simulink library "TYPEA_MASTER"  (Simulink 8.6)
settings: Solver=ode45  StartTime=0.0  StopTime=10.0  RelTol=1e-3
undefined symbols (not defined in the file): CRYP_OLSERVO, PAY_OLSERVO
libraries: cdsFilt x12, GAS_MODAL_MASTER x8, cdsEpicsBinIn x6, VIS_LIB x5, cdsEpicsOut x4, BIO_TYPEA_MASTER x3, cdsDacKill x3, ADV_BF_MASTER x2, cdsEpicsStringIn x2, TYPEA_GAS_MODAL_MASTER x2, ISC_common x2, CRYP_IM_MASTER x2
(part 2 of 2)

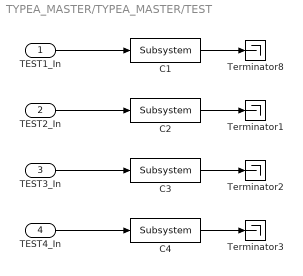
== system TYPEA_MASTER/TYPEA_MASTER/TEST ==
  TEST1_In : Inport
  TEST2_In : Inport  Port=2
  TEST3_In : Inport  Port=3
  TEST4_In : Inport  Port=4
  C1 : cdsFilt/Subsystem  Tag=cdsFilt  Description=|
      | Purpose:                                                                                                                                                                                                                                  
      | Standard CDS IIR filter module.                                                                                                                                                                                                           
      |                                                                                                                                                                                                                                           
      | Operation:                                                                                                                                                                                                                                
      | Consists of 10 second order section IIR filters, plus a ramped gain stage. In FE code, also provides pre-defined test points and excitation channel inputs. The filter coefficients are defined in the LIGO system using the 'foton' tool.
      |                                                                                                                                                                                                                                           
      | Usage:                                                                                                                                                                                                                                    
      | Name the part with the desired filter module name.
      settings: AttributesFormatString=%<Tag>
  C2 : cdsFilt/Subsystem  Tag=cdsFilt  Description=|
      | Purpose:                                                                                                                                                                                                                                  
      | Standard CDS IIR filter module.                                                                                                                                                                                                           
      |                                                                                                                                                                                                                                           
      | Operation:                                                                                                                                                                                                                                
      | Consists of 10 second order section IIR filters, plus a ramped gain stage. In FE code, also provides pre-defined test points and excitation channel inputs. The filter coefficients are defined in the LIGO system using the 'foton' tool.
      |                                                                                                                                                                                                                                           
      | Usage:                                                                                                                                                                                                                                    
      | Name the part with the desired filter module name.
      settings: AttributesFormatString=%<Tag>
  C3 : cdsFilt/Subsystem  Tag=cdsFilt  Description=|
      | Purpose:                                                                                                                                                                                                                                  
      | Standard CDS IIR filter module.                                                                                                                                                                                                           
      |                                                                                                                                                                                                                                           
      | Operation:                                                                                                                                                                                                                                
      | Consists of 10 second order section IIR filters, plus a ramped gain stage. In FE code, also provides pre-defined test points and excitation channel inputs. The filter coefficients are defined in the LIGO system using the 'foton' tool.
      |                                                                                                                                                                                                                                           
      | Usage:                                                                                                                                                                                                                                    
      | Name the part with the desired filter module name.
      settings: AttributesFormatString=%<Tag>
  C4 : cdsFilt/Subsystem  Tag=cdsFilt  Description=|
      | Purpose:                                                                                                                                                                                                                                  
      | Standard CDS IIR filter module.                                                                                                                                                                                                           
      |                                                                                                                                                                                                                                           
      | Operation:                                                                                                                                                                                                                                
      | Consists of 10 second order section IIR filters, plus a ramped gain stage. In FE code, also provides pre-defined test points and excitation channel inputs. The filter coefficients are defined in the LIGO system using the 'foton' tool.
      |                                                                                                                                                                                                                                           
      | Usage:                                                                                                                                                                                                                                    
      | Name the part with the desired filter module name.
      settings: AttributesFormatString=%<Tag>
  Terminator{1..3,8} (4 alike) : Terminator
  wires:
  C2/1 -> Terminator1/1
  C3/1 -> Terminator2/1
  C1/1 -> Terminator8/1
  C4/1 -> Terminator3/1
  TEST1_In/1 -> C1/1
  TEST2_In/1 -> C2/1
  TEST3_In/1 -> C3/1
  TEST4_In/1 -> C4/1

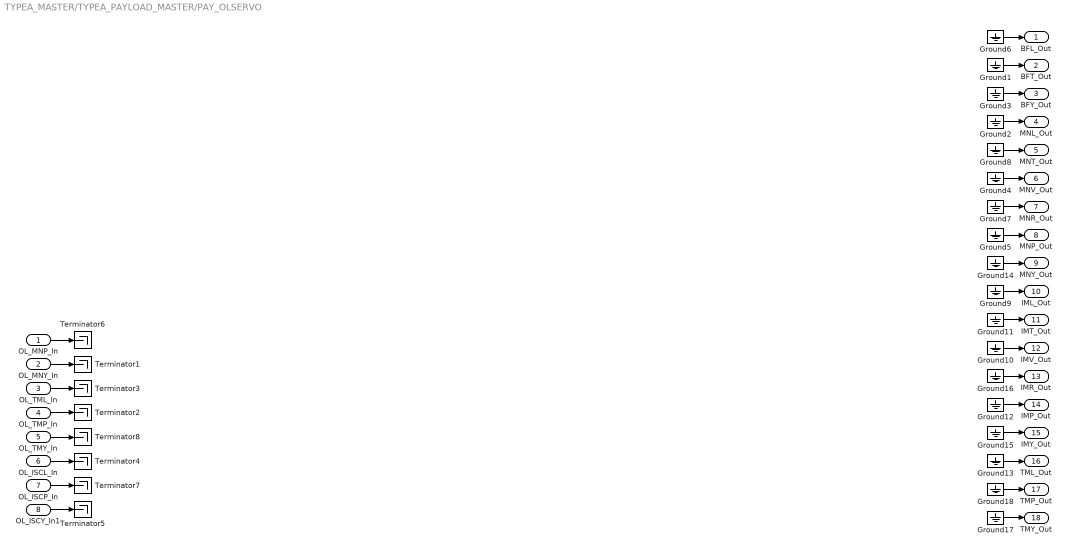
== system TYPEA_MASTER/TYPEA_PAYLOAD_MASTER/PAY_OLSERVO ==
  OL_MNP_In : Inport
  OL_MNY_In : Inport  Port=2
  OL_TML_In : Inport  Port=3
  OL_TMP_In : Inport  Port=4
  OL_TMY_In : Inport  Port=5
  OL_ISCL_In : Inport  Port=6
  OL_ISCP_In : Inport  Port=7
  OL_ISCY_In1 : Inport  Port=8
  Ground{1..18} (18 alike) : Ground
  Terminator{1..8} (8 alike) : Terminator
  BFL_Out : Outport
  BFT_Out : Outport  Port=2
  BFY_Out : Outport  Port=3
  MNL_Out : Outport  Port=4
  MNT_Out : Outport  Port=5
  MNV_Out : Outport  Port=6
  MNR_Out : Outport  Port=7
  MNP_Out : Outport  Port=8
  MNY_Out : Outport  Port=9
  IML_Out : Outport  Port=10
  IMT_Out : Outport  Port=11
  IMV_Out : Outport  Port=12
  IMR_Out : Outport  Port=13
  IMP_Out : Outport  Port=14
  IMY_Out : Outport  Port=15
  TML_Out : Outport  Port=16
  TMP_Out : Outport  Port=17
  TMY_Out : Outport  Port=18
  wires:
  Ground6/1 -> BFL_Out/1
  OL_MNP_In/1 -> Terminator6/1
  OL_MNY_In/1 -> Terminator1/1
  OL_TML_In/1 -> Terminator3/1
  OL_TMP_In/1 -> Terminator2/1
  OL_TMY_In/1 -> Terminator8/1
  OL_ISCL_In/1 -> Terminator4/1
  OL_ISCP_In/1 -> Terminator7/1
  OL_ISCY_In1/1 -> Terminator5/1
  Ground1/1 -> BFT_Out/1
  Ground3/1 -> BFY_Out/1
  Ground2/1 -> MNL_Out/1
  Ground8/1 -> MNT_Out/1
  Ground4/1 -> MNV_Out/1
  Ground7/1 -> MNR_Out/1
  Ground5/1 -> MNP_Out/1
  Ground14/1 -> MNY_Out/1
  Ground9/1 -> IML_Out/1
  Ground11/1 -> IMT_Out/1
  Ground10/1 -> IMV_Out/1
  Ground16/1 -> IMR_Out/1
  Ground12/1 -> IMP_Out/1
  Ground15/1 -> IMY_Out/1
  Ground13/1 -> TML_Out/1
  Ground18/1 -> TMP_Out/1
  Ground17/1 -> TMY_Out/1

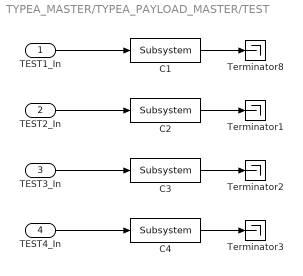
== system TYPEA_MASTER/TYPEA_PAYLOAD_MASTER/TEST ==
  TEST1_In : Inport
  TEST2_In : Inport  Port=2
  TEST3_In : Inport  Port=3
  TEST4_In : Inport  Port=4
  C1 : cdsFilt/Subsystem  Tag=cdsFilt  Description=|
      | Purpose:                                                                                                                                                                                                                                  
      | Standard CDS IIR filter module.                                                                                                                                                                                                           
      |                                                                                                                                                                                                                                           
      | Operation:                                                                                                                                                                                                                                
      | Consists of 10 second order section IIR filters, plus a ramped gain stage. In FE code, also provides pre-defined test points and excitation channel inputs. The filter coefficients are defined in the LIGO system using the 'foton' tool.
      |                                                                                                                                                                                                                                           
      | Usage:                                                                                                                                                                                                                                    
      | Name the part with the desired filter module name.
      settings: AttributesFormatString=%<Tag>
  C2 : cdsFilt/Subsystem  Tag=cdsFilt  Description=|
      | Purpose:                                                                                                                                                                                                                                  
      | Standard CDS IIR filter module.                                                                                                                                                                                                           
      |                                                                                                                                                                                                                                           
      | Operation:                                                                                                                                                                                                                                
      | Consists of 10 second order section IIR filters, plus a ramped gain stage. In FE code, also provides pre-defined test points and excitation channel inputs. The filter coefficients are defined in the LIGO system using the 'foton' tool.
      |                                                                                                                                                                                                                                           
      | Usage:                                                                                                                                                                                                                                    
      | Name the part with the desired filter module name.
      settings: AttributesFormatString=%<Tag>
  C3 : cdsFilt/Subsystem  Tag=cdsFilt  Description=|
      | Purpose:                                                                                                                                                                                                                                  
      | Standard CDS IIR filter module.                                                                                                                                                                                                           
      |                                                                                                                                                                                                                                           
      | Operation:                                                                                                                                                                                                                                
      | Consists of 10 second order section IIR filters, plus a ramped gain stage. In FE code, also provides pre-defined test points and excitation channel inputs. The filter coefficients are defined in the LIGO system using the 'foton' tool.
      |                                                                                                                                                                                                                                           
      | Usage:                                                                                                                                                                                                                                    
      | Name the part with the desired filter module name.
      settings: AttributesFormatString=%<Tag>
  C4 : cdsFilt/Subsystem  Tag=cdsFilt  Description=|
      | Purpose:                                                                                                                                                                                                                                  
      | Standard CDS IIR filter module.                                                                                                                                                                                                           
      |                                                                                                                                                                                                                                           
      | Operation:                                                                                                                                                                                                                                
      | Consists of 10 second order section IIR filters, plus a ramped gain stage. In FE code, also provides pre-defined test points and excitation channel inputs. The filter coefficients are defined in the LIGO system using the 'foton' tool.
      |                                                                                                                                                                                                                                           
      | Usage:                                                                                                                                                                                                                                    
      | Name the part with the desired filter module name.
      settings: AttributesFormatString=%<Tag>
  Terminator{1..3,8} (4 alike) : Terminator
  wires:
  C2/1 -> Terminator1/1
  C3/1 -> Terminator2/1
  C1/1 -> Terminator8/1
  C4/1 -> Terminator3/1
  TEST1_In/1 -> C1/1
  TEST2_In/1 -> C2/1
  TEST3_In/1 -> C3/1
  TEST4_In/1 -> C4/1

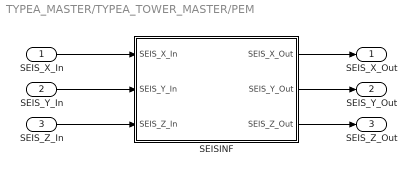
== system TYPEA_MASTER/TYPEA_TOWER_MASTER/PEM ==
  SEIS_X_In : Inport
  SEIS_Y_In : Inport  Port=2
  SEIS_Z_In : Inport  Port=3
  SEISINF : Subsystem
  SEIS_X_Out : Outport
  SEIS_Y_Out : Outport  Port=2
  SEIS_Z_Out : Outport  Port=3
  wires:
  SEIS_X_In/1 -> SEISINF/1(SEIS_X_In)
  SEIS_Y_In/1 -> SEISINF/2(SEIS_Y_In)
  SEIS_Z_In/1 -> SEISINF/3(SEIS_Z_In)
  SEISINF/2(SEIS_Y_Out) -> SEIS_Y_Out/1
  SEISINF/3(SEIS_Z_Out) -> SEIS_Z_Out/1
  SEISINF/1(SEIS_X_Out) -> SEIS_X_Out/1

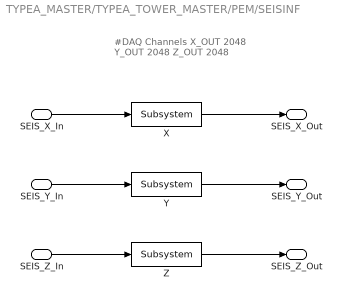
== system TYPEA_MASTER/TYPEA_TOWER_MASTER/PEM/SEISINF ==
  note: #DAQ Channels
      |
      | X_OUT 2048
      | Y_OUT 2048
      | Z_OUT 2048
  SEIS_X_In : Inport
  SEIS_Y_In : Inport  Port=2
  SEIS_Z_In : Inport  Port=3
  X : cdsFilt/Subsystem  Tag=cdsFilt  Description=|
      | Purpose:                                                                                                                                                                                                                                  
      | Standard CDS IIR filter module.                                                                                                                                                                                                           
      |                                                                                                                                                                                                                                           
      | Operation:                                                                                                                                                                                                                                
      | Consists of 10 second order section IIR filters, plus a ramped gain stage. In FE code, also provides pre-defined test points and excitation channel inputs. The filter coefficients are defined in the LIGO system using the 'foton' tool.
      |                                                                                                                                                                                                                                           
      | Usage:                                                                                                                                                                                                                                    
      | Name the part with the desired filter module name.
      settings: AttributesFormatString=%<Tag>
  Y : cdsFilt/Subsystem  Tag=cdsFilt  Description=|
      | Purpose:                                                                                                                                                                                                                                  
      | Standard CDS IIR filter module.                                                                                                                                                                                                           
      |                                                                                                                                                                                                                                           
      | Operation:                                                                                                                                                                                                                                
      | Consists of 10 second order section IIR filters, plus a ramped gain stage. In FE code, also provides pre-defined test points and excitation channel inputs. The filter coefficients are defined in the LIGO system using the 'foton' tool.
      |                                                                                                                                                                                                                                           
      | Usage:                                                                                                                                                                                                                                    
      | Name the part with the desired filter module name.
      settings: AttributesFormatString=%<Tag>
  Z : cdsFilt/Subsystem  Tag=cdsFilt  Description=|
      | Purpose:                                                                                                                                                                                                                                  
      | Standard CDS IIR filter module.                                                                                                                                                                                                           
      |                                                                                                                                                                                                                                           
      | Operation:                                                                                                                                                                                                                                
      | Consists of 10 second order section IIR filters, plus a ramped gain stage. In FE code, also provides pre-defined test points and excitation channel inputs. The filter coefficients are defined in the LIGO system using the 'foton' tool.
      |                                                                                                                                                                                                                                           
      | Usage:                                                                                                                                                                                                                                    
      | Name the part with the desired filter module name.
      settings: AttributesFormatString=%<Tag>
  SEIS_X_Out : Outport
  SEIS_Y_Out : Outport  Port=2
  SEIS_Z_Out : Outport  Port=3
  wires:
  Z/1 -> SEIS_Z_Out/1
  Y/1 -> SEIS_Y_Out/1
  X/1 -> SEIS_X_Out/1
  SEIS_Z_In/1 -> Z/1
  SEIS_X_In/1 -> X/1
  SEIS_Y_In/1 -> Y/1
